simulink model "SPERTE_printer_RC"  (R2024b)
settings: Solver=FixedStepDiscrete  StartTime=0.0  StopTime=tsim  FixedStep=Ts  RelTol=1e-3  EnableMultiTasking=on
InitFcn:
  | Fs = 1000; Ts = 1/Fs;tsim = Inf;
values from neighbouring files (symbols this model uses):
  N = length(r)    [SimExpRC_SPERTE.m]
  N_RC_activate = 5    [SimExpRC_SPERTE.m]
  N_trial = 50    [SimExpRC_SPERTE.m]
  p_Q = M    (= 50)    [DesignControllerRC.m]
undefined symbols (not defined in the file or in its folder): DiscIntNeverNeededParam, p_L
libraries: simulink x7, sperte_lib x3, cstblocks x2
(part 2 of 2)

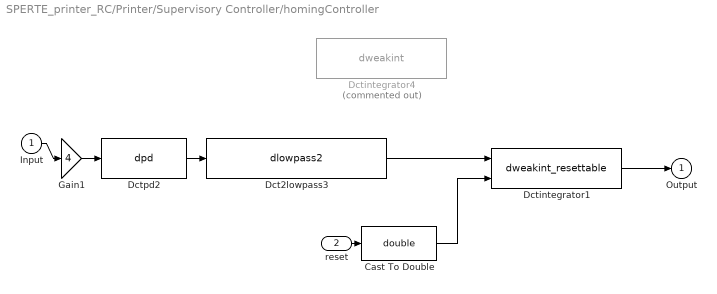
== system SPERTE_printer_RC/Printer/Supervisory Controller/homingController ==
  Input : Inport
  reset : Inport  Port=2
  Cast To Double : DataTypeConversion  OutDataTypeStr=double  SaturateOnIntegerOverflow=off  RndMeth=Floor
  Dct2lowpass3 : S-Function  FunctionName=dlowpass2  Parameters=f_den, b_den, 0.001  SFunctionDeploymentMode=off  EnableBusSupport=off  mask(dctools){f_den=40, b_den=0.7}
      mask prompts: f_den "Pole [Hz]"; b_den "Damping pole [-]"
      mask help: This block implements a discrete time 2nd order lowpass filter.
      mask Display: disp('DCT 2nd order lowpass')
  Dctintegrator1 : S-Function  FunctionName=dweakint_resettable  Parameters=f_num, 0.001  SFunctionDeploymentMode=off  EnableBusSupport=off  mask(dctools){f_num=0.25}
      mask prompts: f_num "Zero [Hz]"
      mask help: This block implements a discrete time weak integrator filter.
      mask Display: disp('DCT integrator')
  Dctintegrator4 : S-Function  Commented=on  FunctionName=dweakint  Parameters=f_num, 0.001  SFunctionDeploymentMode=off  EnableBusSupport=off  mask(dctools){f_num=0.25}
      mask prompts: f_num "Zero [Hz]"
      mask help: This block implements a discrete time weak integrator filter.
      mask Display: disp('DCT integrator')
  Dctpd2 : S-Function  FunctionName=dpd  Parameters=kp, kv, 0.001  SFunctionDeploymentMode=off  EnableBusSupport=off  mask(dctools){kp=40, kv=1}
      mask help: This block implements a discrete time pd filter.
      mask Display: disp('DCT pd')
  Gain1 : Gain  Gain=4  SaturateOnIntegerOverflow=on  OutDataTypeStr=Inherit: Same as input  ParamDataTypeStr=Inherit: Same as input
  Output : Outport
  wires:
  Input/1 -> Gain1/1
  Gain1/1 -> Dctpd2/1
  Dctpd2/1 -> Dct2lowpass3/1
  Dctintegrator1/1 -> Output/1
  Cast To Double/1 -> Dctintegrator1/2
  Dct2lowpass3/1 -> Dctintegrator1/1
  reset/1 -> Cast To Double/1

== stateflow chart SPERTE_printer_RC/Printer/Supervisory Controller/Supervisor ==
  state AirbagLeft
    entry:
    airBagEnabled = 1;
    airBagRef=-0.01;
  state DisableOutputs
    entry:
    controlEnabled=0;
  state Homing
    entry:
    %Set jog speed and homing state
    toPoint = 0;
    homingBusy = 1;
    jogSpeed = -0.2;
    homeControllerEnabled=1;
  state AirbagRight
    entry:
    airBagEnabled = 1;
    airBagRef=0.35;
  state EnableRunAndSafety
    entry:
    resetEnc=0;
    homingBusy=0;
  state MovetoX0
    entry:
    jogSpeed = 0.0;
    toPoint = 0.06;
  state ResetEnc
    entry:
    resetEnc=1;
  state DisableControl
    entry:
    homeControllerEnabled=0;
  (default) -> Homing
  AirbagLeft -> DisableOutputs : after(1,sec)
  AirbagRight -> DisableOutputs : after(1,sec)
  EnableRunAndSafety -> Homing [order 1] : [reset_homing]
  EnableRunAndSafety -> AirbagLeft [order 2] : [carPos<-0.01]
  Homing -> MovetoX0 : %Transition if homeswitch becomes high
      | [homeSwitch]
  EnableRunAndSafety -> AirbagRight [order 3] : [carPos>0.35]
  ResetEnc -> EnableRunAndSafety : after(0.1,sec)
  MovetoX0 -> DisableControl : %Allow time for moving
      | after(1,sec)
  DisableControl -> ResetEnc : %Allow settling of belt
      | after(0.5,sec)
  data: jogSpeed output double; toPoint output double; homeControllerEnabled output double; resetEnc output double; homingBusy output double =1; homeSwitch input double; carPos input double; airBagEnabled output double =0; airBagRef output double =0; controlEnabled output double =1; reset_homing input; SupervisorMode output Enum: SupervisorModeType
